simulink model "untitled_restored_from_autosave"  (R2022a)
settings: Solver=VariableStepAuto  StartTime=0.0  StopTime=15  RelTol=1e-3
settings Model: Creator=sarah  LastModifiedBy=sarah

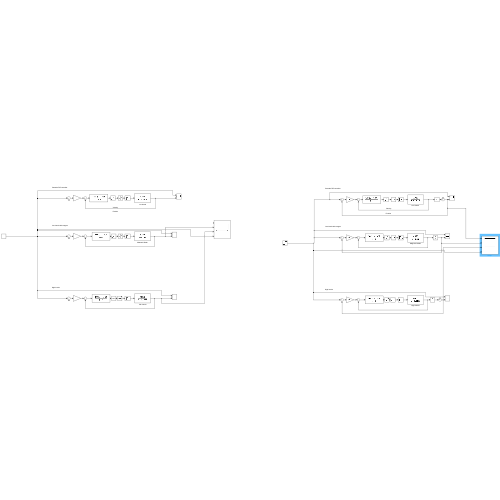
[thumbnail: Simulink's stored preview of the top-level diagram]
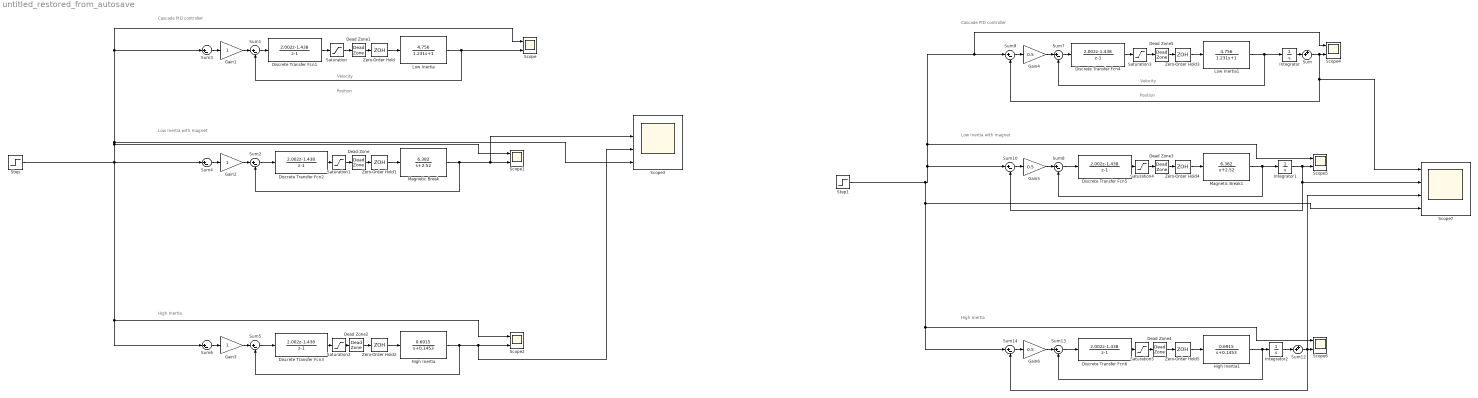
== system untitled_restored_from_autosave ==
  note: Position
  note: Cascade PID controller
  note: Low Inertia with magnet
  note: Velocity
  note: High Inertia
  note: Cascade PID controller
  note: Velocity
  note: Low Inertia with magnet
  note: High Inertia
  note: Position
  Dead Zone : DeadZone  LowerValue=-1.53  UpperValue=0.39
  Dead Zone1 : DeadZone  LowerValue=-1.48  UpperValue=00.39
  Dead Zone2 : DeadZone  LowerValue=-0.49  UpperValue=0.43
  Dead Zone3 : DeadZone  LowerValue=-1.53  UpperValue=0.39
  Dead Zone4 : DeadZone  LowerValue=-0.49  UpperValue=0.43
  Dead Zone5 : DeadZone  LowerValue=-1.48  UpperValue=00.39
  Discrete Transfer Fcn{1..6} (6 alike) : DiscreteTransferFcn  Numerator=[2.002 -1.438]  Denominator=[1 -1]  SampleTime=0.05
  Gain1 : Gain
  Gain2 : Gain
  Gain3 : Gain
  Gain4 : Gain  Gain=0.5
  Gain5 : Gain  Gain=0.5
  Gain6 : Gain  Gain=0.5
  High Inertia : TransferFcn  Numerator=[0.6915]  Denominator=[1 0.1453]
  High Inertia1 : TransferFcn  Numerator=[0.6915]  Denominator=[1 0.1453]
  Integrator : Integrator
  Integrator1 : Integrator
  Integrator2 : Integrator
  Low Inertia : TransferFcn  Numerator=[4.756]  Denominator=[1.231 1]
  Low Inertia1 : TransferFcn  Numerator=[4.756]  Denominator=[1.231 1]
  Magnetic Break : TransferFcn  Numerator=[6.382]  Denominator=[1 2.52]
  Magnetic Break1 : TransferFcn  Numerator=[6.382]  Denominator=[1 2.52]
  Saturation{,1..5} (6 alike) : Saturate  UpperLimit=+10  LowerLimit=-10
  Scope : Scope  NumInputPorts=3
  Scope1 : Scope  NumInputPorts=3
  Scope2 : Scope  NumInputPorts=3
  Scope3 : Scope  NumInputPorts=4
  Scope4 : Scope  NumInputPorts=2
  Scope5 : Scope  NumInputPorts=2
  Scope6 : Scope  NumInputPorts=2
  Scope7 : Scope  NumInputPorts=4
  Step : Step  Time=0  After=5  SampleTime=0
  Step1 : Step  Time=0  After=5  SampleTime=0
  Sum : Sum  Inputs=++|
  Sum{1..10,13..14} (12 alike) : Sum  Inputs=|+-
  Sum12 : Sum  Inputs=++|
  Zero-Order Hold{,1,3..4} (4 alike) : ZeroOrderHold  SampleTime=0.05
  Zero-Order Hold2 : ZeroOrderHold  SampleTime=0.02
  Zero-Order Hold5 : ZeroOrderHold  SampleTime=0.02
  wires:
  Dead Zone/1 -> Zero-Order Hold1/1
  Saturation1/1 -> Dead Zone/1
  Sum3/1 -> Gain1/1
  Zero-Order Hold/1 -> Low Inertia/1
  High Inertia/1 -> Scope3/3, Scope2/3, Sum5/2
  Sum1/1 -> Discrete Transfer Fcn1/1
  Discrete Transfer Fcn3/1 -> Saturation2/1
  Discrete Transfer Fcn1/1 -> Saturation/1
  Sum5/1 -> Discrete Transfer Fcn3/1
  Gain2/1 -> Sum2/1
  Zero-Order Hold1/1 -> Magnetic Break/1
  Sum2/1 -> Discrete Transfer Fcn2/1
  Sum4/1 -> Gain2/1
  Magnetic Break/1 -> Scope3/2, Scope1/3, Sum2/2
  Step/1 -> Sum4/1, Scope2/1, Sum6/1, Scope1/1, Scope/1, Sum3/1, Scope3/4
  Sum6/1 -> Gain3/1
  Discrete Transfer Fcn2/1 -> Saturation1/1
  Zero-Order Hold2/1 -> High Inertia/1
  Gain1/1 -> Sum1/1
  Gain3/1 -> Sum5/1
  Low Inertia/1 -> Scope/3, Sum1/2
  Dead Zone2/1 -> Zero-Order Hold2/1
  Saturation2/1 -> Dead Zone2/1
  Saturation/1 -> Dead Zone1/1
  Dead Zone1/1 -> Zero-Order Hold/1
  Sum7/1 -> Discrete Transfer Fcn4/1
  Saturation4/1 -> Dead Zone3/1
  Dead Zone3/1 -> Zero-Order Hold4/1
  Saturation5/1 -> Dead Zone4/1
  Sum/1 -> Scope7/1, Sum9/2, Scope4/2
  Integrator/1 -> Sum/2
  Discrete Transfer Fcn6/1 -> Saturation5/1
  Gain4/1 -> Sum7/1
  Integrator2/1 -> Sum12/2
  Zero-Order Hold3/1 -> Low Inertia1/1
  Sum12/1 -> Sum14/2, Scope7/3, Scope6/2
  Sum13/1 -> Discrete Transfer Fcn6/1
  Saturation3/1 -> Dead Zone5/1
  Low Inertia1/1 -> Integrator/1, Sum7/2
  Discrete Transfer Fcn5/1 -> Saturation4/1
  Zero-Order Hold5/1 -> High Inertia1/1
  Magnetic Break1/1 -> Sum8/2, Integrator1/1
  Sum8/1 -> Discrete Transfer Fcn5/1
  High Inertia1/1 -> Sum13/2, Integrator2/1
  Sum14/1 -> Gain6/1
  Sum9/1 -> Gain4/1
  Dead Zone5/1 -> Zero-Order Hold3/1
  Zero-Order Hold4/1 -> Magnetic Break1/1
  Dead Zone4/1 -> Zero-Order Hold5/1
  Gain5/1 -> Sum8/1
  Sum10/1 -> Gain5/1
  Gain6/1 -> Sum13/1
  Discrete Transfer Fcn4/1 -> Saturation3/1
  Integrator1/1 -> Sum10/2, Scope7/2, Scope5/2
  Step1/1 -> Scope6/1, Sum14/1, Scope7/4, Scope5/1, Scope4/1, Sum9/1, Sum10/1
